simulink model "regulator_ze_sprzezeniem_od_stanu"  (R2018b)
settings: Solver=VariableStepAuto  StartTime=0.0  StopTime=10  RelTol=1e-3
values from neighbouring files (symbols this model uses):
  K_x = K_9    [zad5.m]
undefined symbols (not defined in the file or in its folder): A, C
settings Model: Creator=mariu  LastModifiedBy=mariu

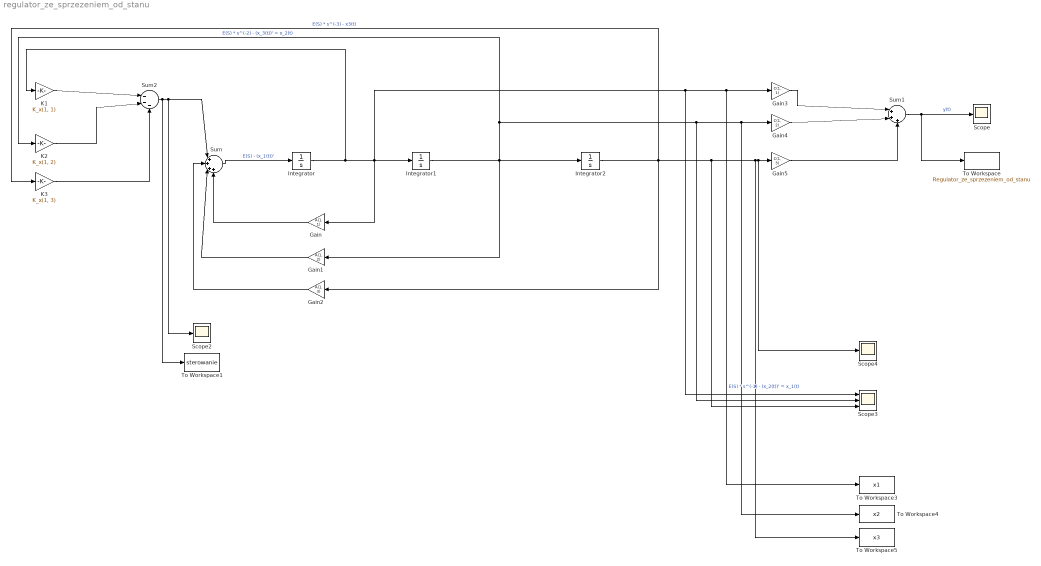
== system regulator_ze_sprzezeniem_od_stanu ==
  Gain : Gain  Gain=A(1, 1)
  Gain1 : Gain  Gain=A(1, 2)
  Gain2 : Gain  Gain=A(1, 3)
  Gain3 : Gain  Gain=C(1, 1)
  Gain4 : Gain  Gain=C(1, 2)
  Gain5 : Gain  Gain=C(1, 3)
  Integrator : Integrator  InitialCondition=-1
  Integrator1 : Integrator  InitialCondition=2
  Integrator2 : Integrator  InitialCondition=1
  "K1 " : Gain  Gain=K_x(1, 1)
  "K2 " : Gain  Gain=K_x(1, 2)
  "K3 " : Gain  Gain=K_x(1, 3)
  Scope : Scope
  Scope2 : Scope
  Scope3 : Scope  NumInputPorts=3
  Scope4 : Scope
  Sum : Sum  Inputs=|++++
      settings: AttributesFormatString=%<Inputs>
  Sum1 : Sum  Inputs=|+++
      settings: AttributesFormatString=%<Inputs>
  Sum2 : Sum  Inputs=|---
      settings: AttributesFormatString=%<Inputs>
  To Workspace : ToWorkspace  VariableName=Regulator_ze_sprzezeniem_od_stanu  SaveFormat=Timeseries  SampleTime=-1
  To Workspace1 : ToWorkspace  VariableName=sterowanie  SaveFormat=Timeseries  SampleTime=-1
  To Workspace3 : ToWorkspace  VariableName=x1  SaveFormat=Timeseries  SampleTime=-1
  To Workspace4 : ToWorkspace  VariableName=x2  SaveFormat=Timeseries  SampleTime=-1
  To Workspace5 : ToWorkspace  VariableName=x3  SaveFormat=Timeseries  SampleTime=-1
  wires:
  Sum1/1 -> To Workspace/1, Scope/1  "y(t)"
  Integrator1/1 -> "K2 "/1, Scope3/2, To Workspace4/1, Gain4/1, Gain1/1, Integrator2/1  "E(S) * s^(-2) - (x_3(t))' = x_2(t)"
  Gain3/1 -> Sum1/1
  Integrator/1 -> "K1 "/1, Scope3/1, To Workspace3/1, Gain3/1, Gain/1, Integrator1/1  "E(S) * s^(-1) - (x_2(t))' = x_1(t)"
  Gain5/1 -> Sum1/3
  Sum/1 -> Integrator/1  "E(S) - (x_1(t))'"
  Integrator2/1 -> Gain2/1, "K3 "/1, Scope3/3, Scope4/1, Gain5/1, To Workspace5/1  "E(S) * s^(-3) - x3(t)"
  Gain4/1 -> Sum1/2
  Gain1/1 -> Sum/3
  Gain/1 -> Sum/4
  Gain2/1 -> Sum/2
  "K2 "/1 -> Sum2/2
  "K1 "/1 -> Sum2/1
  "K3 "/1 -> Sum2/3
  Sum2/1 -> To Workspace1/1, Scope2/1, Sum/1
